simulink model "SimulationEchantillinnesClampingMCC_Simplified"  (R2018b)
settings: Solver=VariableStepAuto  StartTime=0.0  StopTime=2  MaxStep=Ts_elec  RelTol=1e-3
values from neighbouring files (symbols this model uses):
  Imax = Inom    (= 4.4)    [DataMCCEchant.m]
  Kelec = -place(Ae,Be,Pole_elec_desiree)    [DataMCCEchant.m]
  Kmeca = place(Am,Bm,Pole_meca_desiree)    [DataMCCEchant.m]
  Vmax = Vdc    (= 24)    [DataMCCEchant.m]
undefined symbols (not defined in the file or in its folder): DiscIntNeverNeededParam
libraries: simulink x3
settings Model: Creator=romaindelpoux  LastModifiedBy=rdelpoux
settings SolverCC: ZeroCrossControl=DisableAll  AlgebraicLoopSolver=LineSearch
settings SFSimCC: SimUseLocalCustomCode=off
settings RTWCC: RTWUseLocalCustomCode=off

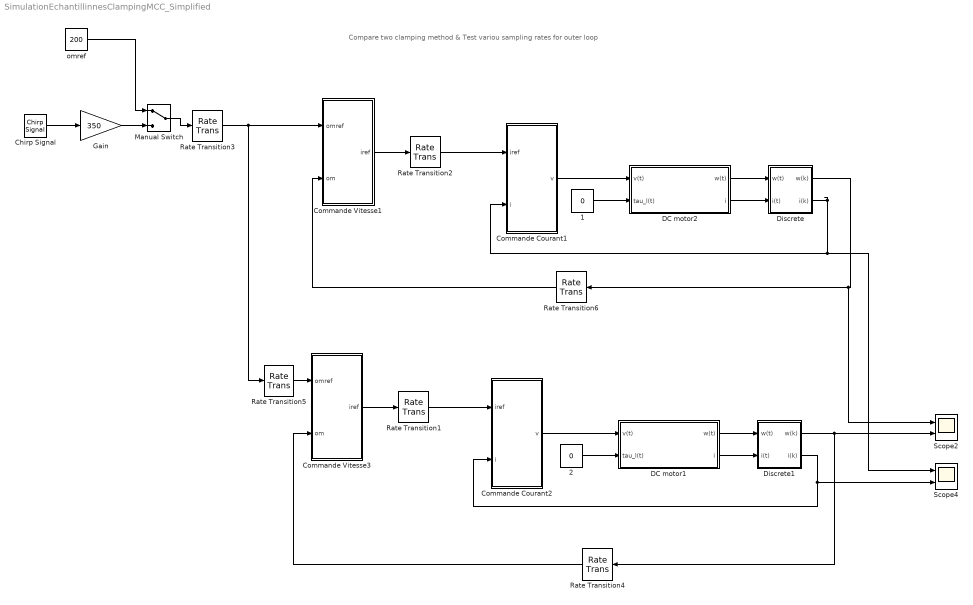
== system SimulationEchantillinnesClampingMCC_Simplified ==
  note: Compare two clamping method
      | & Test variou sampling rates for outer loop
  " 2" : Constant  Value=0
  1 : Constant  Value=0
  Chirp Signal : simulink/Sources/Chirp Signal  f1=0.1  T=20  f2=5
  Commande Courant1 : Subsystem
  Commande Courant2 : Subsystem
  Commande Vitesse1 : Subsystem
  Commande Vitesse3 : Subsystem
  DC motor1 : Subsystem  mask{R=1.22, L=0.0027, Kphi=0.061, J=0.22e-3, F=.0001, C0=0}
      mask prompts: R "Resistance (R) in Ohms"; L "Inductance (L) in H"; Kphi "Back EMF (Kphi) in V/rad/s"; J "J in kgm²"; F "F in N/rad/s"
      mask DialogControl Container3 Prompt: Electrical Parameters
      mask DialogControl Container3_copy Prompt: Mechanical Parameters
  DC motor2 : Subsystem  mask{R=1.22, L=0.0027, Kphi=0.061, J=0.22e-3, F=.0001, C0=0}
      mask prompts: R "Resistance (R) in Ohms"; L "Inductance (L) in H"; Kphi "Back EMF (Kphi) in V/rad/s"; J "J in kgm²"; F "F in N/rad/s"
      mask DialogControl Container3 Prompt: Electrical Parameters
      mask DialogControl Container3_copy Prompt: Mechanical Parameters
  Discrete : Subsystem
  Discrete1 : Subsystem
  Gain : Gain  Gain=350  OutDataTypeStr=Inherit: Inherit via back propagation
  Manual Switch : ManualSwitch
  Rate Transition1 : RateTransition  Deterministic=off  OutPortSampleTime=50e-6
  Rate Transition2 : RateTransition  Deterministic=off  OutPortSampleTime=50e-6
  Rate Transition3 : RateTransition  Deterministic=off  OutPortSampleTime=.002
  Rate Transition4 : RateTransition  Deterministic=off  OutPortSampleTime=0.002
  Rate Transition5 : RateTransition  Deterministic=off
  Rate Transition6 : RateTransition  Deterministic=off  OutPortSampleTime=0.002
  Scope2 : Scope  NumInputPorts=2
  Scope4 : Scope  NumInputPorts=2
  omref : Constant  Value=200  OutDataTypeStr=Inherit: Inherit via back propagation
  wires:
  Chirp Signal/1 -> Gain/1
  Rate Transition2/1 -> Commande Courant1/1(iref)
  DC motor2/1(w(t)) -> Discrete/1(w(t))
  DC motor2/2(i) -> Discrete/2(i(t))
  Discrete/1(w(k)) -> Scope2/1, Rate Transition6/1
  1/1 -> DC motor2/2(tau_l(t))
  Commande Vitesse1/1(iref) -> Rate Transition2/1
  Commande Courant1/1(v) -> DC motor2/1(v(t))
  Gain/1 -> Manual Switch/2
  Manual Switch/1 -> Rate Transition3/1
  omref/1 -> Manual Switch/1
  Rate Transition3/1 -> Rate Transition5/1, Commande Vitesse1/1(omref)
  Commande Courant2/1(v) -> DC motor1/1(v(t))
  Commande Vitesse3/1(iref) -> Rate Transition1/1
  " 2"/1 -> DC motor1/2(tau_l(t))
  Discrete1/1(w(k)) -> Scope2/2, Rate Transition4/1
  DC motor1/1(w(t)) -> Discrete1/1(w(t))
  DC motor1/2(i) -> Discrete1/2(i(t))
  Rate Transition1/1 -> Commande Courant2/1(iref)
  Discrete1/2(i(k)) -> Scope4/2, Commande Courant2/2(i)
  Rate Transition5/1 -> Commande Vitesse3/1(omref)
  Rate Transition4/1 -> Commande Vitesse3/2(om)
  Discrete/2(i(k)) -> Scope4/1, Commande Courant1/2(i)
  Rate Transition6/1 -> Commande Vitesse1/2(om)

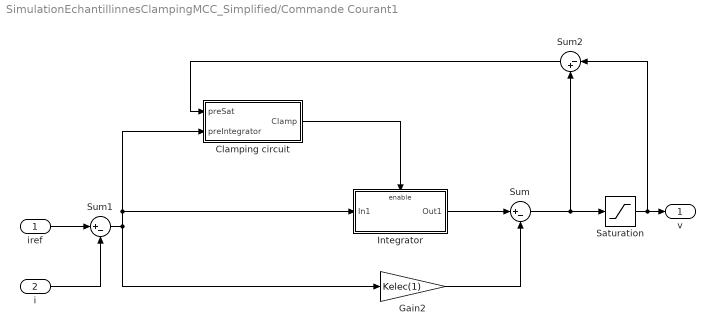
== system SimulationEchantillinnesClampingMCC_Simplified/Commande Courant1 ==
  iref : Inport
  i : Inport  Port=2
  Clamping circuit : Subsystem
  Gain2 : Gain  Gain=Kelec(1)
  Integrator : Subsystem
  Saturation : Saturate  UpperLimit=Vmax  LowerLimit=-Vmax
  Sum : Sum  Inputs=|+-
  Sum1 : Sum  Inputs=|+-
  Sum2 : Sum  Inputs=|-+  OutDataTypeStr=Inherit: Same as accumulator
  v : Outport
  wires:
  Gain2/1 -> Sum/2
  i/1 -> Sum1/2
  iref/1 -> Sum1/1
  Sum1/1 -> Clamping circuit/2(preIntegrator), Integrator/1(In1), Gain2/1
  Clamping circuit/1(Clamp) -> Integrator/Enable
  Sum/1 -> Sum2/2, Saturation/1
  Sum2/1 -> Clamping circuit/1(preSat)
  Saturation/1 -> Sum2/1, v/1
  Integrator/1(Out1) -> Sum/1

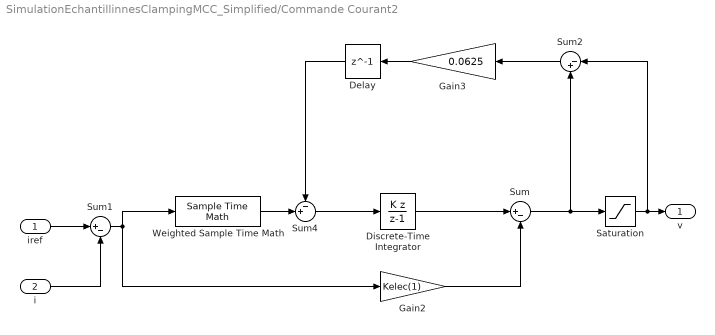
== system SimulationEchantillinnesClampingMCC_Simplified/Commande Courant2 ==
  iref : Inport
  i : Inport  Port=2
  Delay : Delay  DelayLength=1  InitialCondition=0
  Discrete-Time Integrator : DiscreteIntegrator  IntegratorMethod=Accumulation: Backward Euler  SampleTime=-1  ICPrevOutput=DiscIntNeverNeededParam  ICPrevScaledInput=DiscIntNeverNeededParam
  Gain2 : Gain  Gain=Kelec(1)
  Gain3 : Gain  Gain=0.0625
  Saturation : Saturate  UpperLimit=Vmax  LowerLimit=-Vmax
  Sum : Sum  Inputs=|+-
  Sum1 : Sum  Inputs=|+-
  Sum2 : Sum  Inputs=|-+  OutDataTypeStr=Inherit: Same as accumulator
  Sum4 : Sum  Inputs=-+|
  Weighted Sample Time Math : SampleTimeMath  TsampMathOp=*  weightValue=Kelec(2)  TsampMathImp=Offline Scaling Adjustment
  v : Outport
  wires:
  Saturation/1 -> v/1, Sum2/1
  Sum/1 -> Saturation/1, Sum2/2
  iref/1 -> Sum1/1
  i/1 -> Sum1/2
  Gain2/1 -> Sum/2
  Sum1/1 -> Gain2/1, Weighted Sample Time Math/1
  Sum4/1 -> Discrete-Time Integrator/1
  Gain3/1 -> Delay/1
  Delay/1 -> Sum4/1
  Discrete-Time Integrator/1 -> Sum/1
  Sum2/1 -> Gain3/1
  Weighted Sample Time Math/1 -> Sum4/2

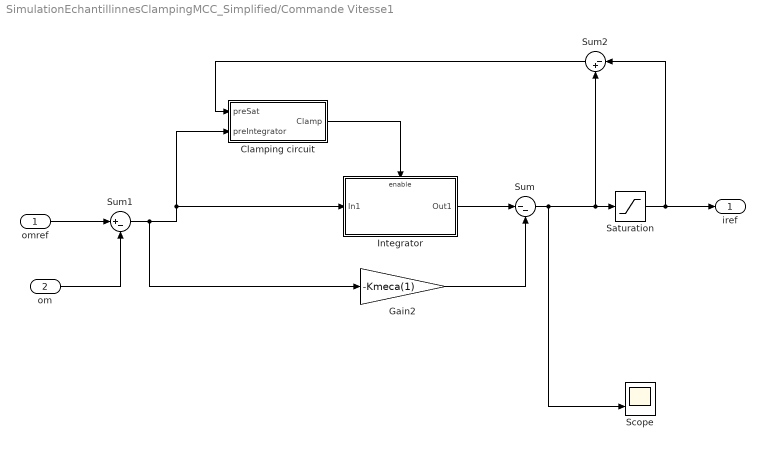
== system SimulationEchantillinnesClampingMCC_Simplified/Commande Vitesse1 ==
  omref : Inport
  om : Inport  Port=2
  Clamping circuit : Subsystem
  Gain2 : Gain  Gain=-Kmeca(1)
  Integrator : Subsystem
  Saturation : Saturate  UpperLimit=Imax  LowerLimit=-Imax
  Scope : Scope  NumInputPorts=2
  Sum : Sum  Inputs=|--
  Sum1 : Sum  Inputs=|+-
  Sum2 : Sum  Inputs=|-+  OutDataTypeStr=Inherit: Same as accumulator
  iref : Outport
  wires:
  Saturation/1 -> Sum2/1, iref/1
  Sum/1 -> Sum2/2, Saturation/1, Scope/2
  om/1 -> Sum1/2
  Gain2/1 -> Sum/2
  omref/1 -> Sum1/1
  Sum2/1 -> Clamping circuit/1(preSat)
  Sum1/1 -> Clamping circuit/2(preIntegrator), Integrator/1(In1), Gain2/1
  Integrator/1(Out1) -> Sum/1
  Clamping circuit/1(Clamp) -> Integrator/Enable

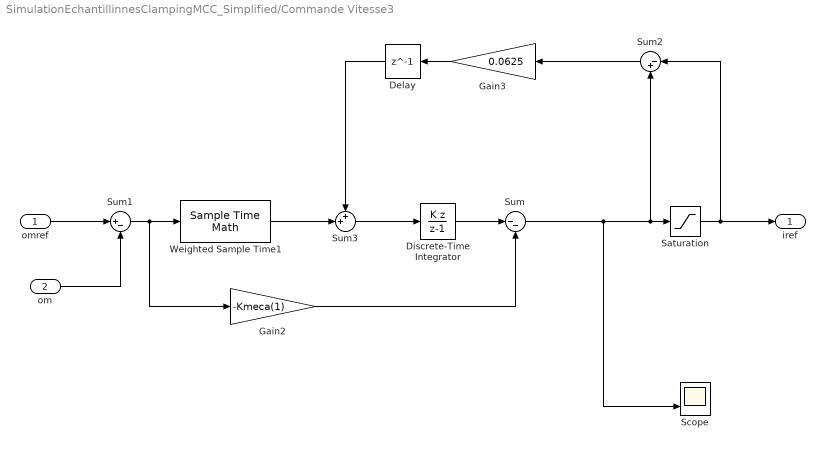
== system SimulationEchantillinnesClampingMCC_Simplified/Commande Vitesse3 ==
  omref : Inport
  om : Inport  Port=2
  Delay : Delay  DelayLength=1  InitialCondition=0
  Discrete-Time Integrator : DiscreteIntegrator  IntegratorMethod=Accumulation: Backward Euler  SampleTime=-1  ICPrevOutput=DiscIntNeverNeededParam  ICPrevScaledInput=DiscIntNeverNeededParam
  Gain2 : Gain  Gain=-Kmeca(1)
  Gain3 : Gain  Gain=0.0625
  Saturation : Saturate  UpperLimit=Imax  LowerLimit=-Imax
  Scope : Scope  NumInputPorts=2
  Sum : Sum  Inputs=|--
  Sum1 : Sum  Inputs=|+-
  Sum2 : Sum  Inputs=|-+  OutDataTypeStr=Inherit: Same as accumulator
  Sum3 : Sum  Inputs=++|
  Weighted Sample Time1 : SampleTimeMath  TsampMathOp=*  weightValue=Kmeca(2)
  iref : Outport
  wires:
  Delay/1 -> Sum3/1
  Gain3/1 -> Delay/1
  Sum3/1 -> Discrete-Time Integrator/1
  Discrete-Time Integrator/1 -> Sum/1
  Saturation/1 -> iref/1, Sum2/1
  Sum/1 -> Scope/2, Sum2/2, Saturation/1
  om/1 -> Sum1/2
  omref/1 -> Sum1/1
  Sum2/1 -> Gain3/1
  Gain2/1 -> Sum/2
  Sum1/1 -> Weighted Sample Time1/1, Gain2/1
  Weighted Sample Time1/1 -> Sum3/2

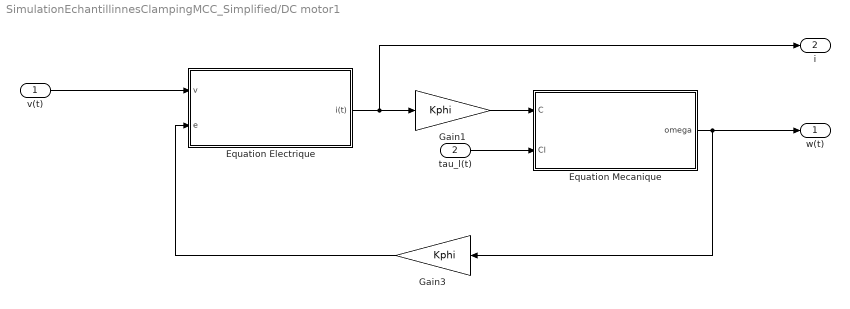
== system SimulationEchantillinnesClampingMCC_Simplified/DC motor1 ==
  v(t) : Inport
  tau_l(t) : Inport  Port=2
  Equation Electrique : Subsystem
  Equation Mecanique : Subsystem
  Gain1 : Gain  Gain=Kphi
  "Gain3  " : Gain  Gain=Kphi
  w(t) : Outport
  i : Outport  Port=2
  wires:
  "Gain3  "/1 -> Equation Electrique/2(e)
  Gain1/1 -> Equation Mecanique/1(C)
  tau_l(t)/1 -> Equation Mecanique/2(Cl)
  Equation Electrique/1(i(t)) -> i/1, Gain1/1
  Equation Mecanique/1(omega) -> w(t)/1, "Gain3  "/1
  v(t)/1 -> Equation Electrique/1(v)

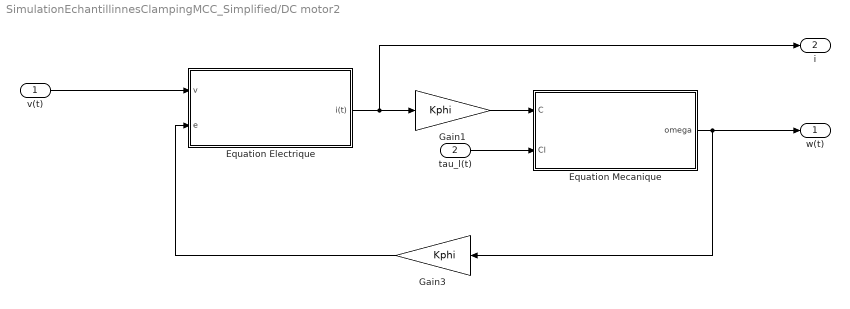
== system SimulationEchantillinnesClampingMCC_Simplified/DC motor2 ==
  v(t) : Inport
  tau_l(t) : Inport  Port=2
  Equation Electrique : Subsystem
  Equation Mecanique : Subsystem
  Gain1 : Gain  Gain=Kphi
  "Gain3  " : Gain  Gain=Kphi
  w(t) : Outport
  i : Outport  Port=2
  wires:
  v(t)/1 -> Equation Electrique/1(v)
  Equation Mecanique/1(omega) -> "Gain3  "/1, w(t)/1
  Equation Electrique/1(i(t)) -> Gain1/1, i/1
  tau_l(t)/1 -> Equation Mecanique/2(Cl)
  Gain1/1 -> Equation Mecanique/1(C)
  "Gain3  "/1 -> Equation Electrique/2(e)

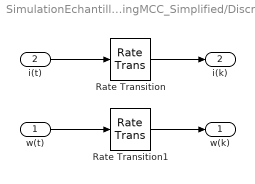
== system SimulationEchantillinnesClampingMCC_Simplified/Discrete ==
  w(t) : Inport
  i(t) : Inport  Port=2
  Rate Transition : RateTransition  Deterministic=off  OutPortSampleTime=50e-6
  Rate Transition1 : RateTransition  Deterministic=off  OutPortSampleTime=.002
  w(k) : Outport
  i(k) : Outport  Port=2
  wires:
  w(t)/1 -> Rate Transition1/1
  i(t)/1 -> Rate Transition/1
  Rate Transition1/1 -> w(k)/1
  Rate Transition/1 -> i(k)/1

== system SimulationEchantillinnesClampingMCC_Simplified/Discrete1 ==
  w(t) : Inport
  i(t) : Inport  Port=2
  Rate Transition : RateTransition  Deterministic=off  OutPortSampleTime=50e-6
  Rate Transition1 : RateTransition  Deterministic=off  OutPortSampleTime=.002
  w(k) : Outport
  i(k) : Outport  Port=2
  wires:
  Rate Transition/1 -> i(k)/1
  Rate Transition1/1 -> w(k)/1
  i(t)/1 -> Rate Transition/1
  w(t)/1 -> Rate Transition1/1

== system SimulationEchantillinnesClampingMCC_Simplified/Commande Courant1/Clamping circuit ==
  note: La logique de clamping permet de bloquer l'entée de l'action intégrale.
      | Ainsi, si la sortie du controlleur est en dehors des limites imposés (saturée), alors l'action intégrale du correcteur est verrouyé (clamping).
      | L'action intégrale est verroullé si la sortie du correcteur (commande) est en dehors des saturations et que le signe de cette sortie est égale
      | à l'entrée du signal à intégrer.
  preSat : Inport  DisableCoverage=on
  preIntegrator : Inport  DisableCoverage=on  Port=2
  Compare To Zero1 : simulink/Logic and Bit Operations/Compare To Zero  relop=<=  OutDataTypeStr=boolean
  Delay : Delay  DelayLength=1  InitialCondition=0
  Multiply : Product
  Clamp : Outport  DisableCoverage=on
  wires:
  Compare To Zero1/1 -> Clamp/1
  preIntegrator/1 -> Multiply/2
  Multiply/1 -> Compare To Zero1/1
  preSat/1 -> Delay/1
  Delay/1 -> Multiply/1

== system SimulationEchantillinnesClampingMCC_Simplified/Commande Courant1/Integrator ==
  In1 : Inport
  Enable : EnablePort
  Discrete-Time Integrator : DiscreteIntegrator  SampleTime=50e-6  ICPrevOutput=DiscIntNeverNeededParam  ICPrevScaledInput=DiscIntNeverNeededParam
  Gain1 : Gain  Gain=Kelec(2)
  Out1 : Outport
  wires:
  Discrete-Time Integrator/1 -> Gain1/1
  In1/1 -> Discrete-Time Integrator/1
  Gain1/1 -> Out1/1

== system SimulationEchantillinnesClampingMCC_Simplified/Commande Vitesse1/Clamping circuit ==
  note: La logique de clamping permet de bloquer l'entée de l'action intégrale.
      | Ainsi, si la sortie du controlleur est en dehors des limites imposés (saturée), alors l'action intégrale du correcteur est verrouyé (clamping).
      | L'action intégrale est verroullé si la sortie du correcteur (commande) est en dehors des saturations et que le signe de cette sortie est égale
      | à l'entrée du signal à intégrer.
  preSat : Inport  DisableCoverage=on
  preIntegrator : Inport  DisableCoverage=on  Port=2
  Compare To Zero1 : simulink/Logic and Bit Operations/Compare To Zero  relop=<=  OutDataTypeStr=boolean
  Delay : Delay  DelayLength=1  InitialCondition=0
  Multiply : Product
  Clamp : Outport  DisableCoverage=on
  wires:
  Compare To Zero1/1 -> Clamp/1
  preIntegrator/1 -> Multiply/2
  Multiply/1 -> Compare To Zero1/1
  preSat/1 -> Delay/1
  Delay/1 -> Multiply/1

== system SimulationEchantillinnesClampingMCC_Simplified/Commande Vitesse1/Integrator ==
  In1 : Inport
  Enable : EnablePort
  Discrete-Time Integrator : DiscreteIntegrator  SampleTime=-1  ICPrevOutput=DiscIntNeverNeededParam  ICPrevScaledInput=DiscIntNeverNeededParam
  Gain1 : Gain  Gain=Kmeca(2)
  Out1 : Outport
  wires:
  Discrete-Time Integrator/1 -> Gain1/1
  Gain1/1 -> Out1/1
  In1/1 -> Discrete-Time Integrator/1

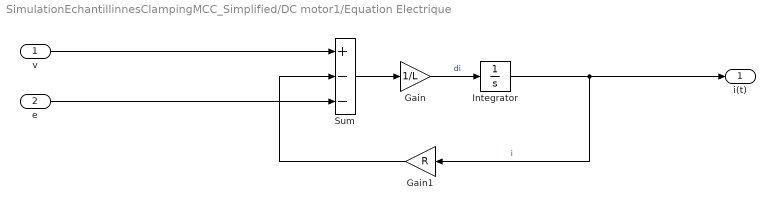
== system SimulationEchantillinnesClampingMCC_Simplified/DC motor1/Equation Electrique ==
  v : Inport
  e : Inport  Port=2
  Gain : Gain  Gain=1/L
  Gain1 : Gain  Gain=R
  Integrator : Integrator
  Sum : Sum  Inputs=+--
  i(t) : Outport
  wires:
  Gain1/1 -> Sum/2
  Sum/1 -> Gain/1
  Integrator/1 -> i(t)/1, Gain1/1  "i"
  Gain/1 -> Integrator/1  "di"
  v/1 -> Sum/1
  e/1 -> Sum/3

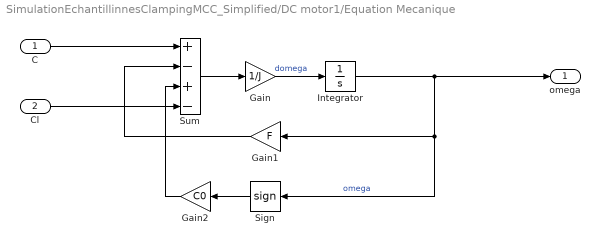
== system SimulationEchantillinnesClampingMCC_Simplified/DC motor1/Equation Mecanique ==
  C : Inport
  Cl : Inport  Port=2
  Gain : Gain  Gain=1/J
  Gain1 : Gain  Gain=F
  Gain2 : Gain  Gain=C0
  Integrator : Integrator
  Sign : Signum
  Sum : Sum  Inputs=+-+-
  omega : Outport
  wires:
  Gain/1 -> Integrator/1  "domega"
  Integrator/1 -> Sign/1, Gain1/1, omega/1  "omega"
  Sum/1 -> Gain/1
  Gain1/1 -> Sum/2
  Sign/1 -> Gain2/1
  Gain2/1 -> Sum/3
  C/1 -> Sum/1
  Cl/1 -> Sum/4

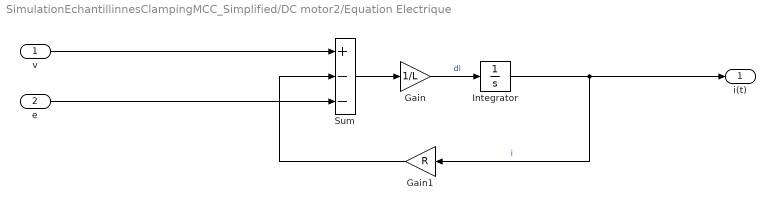
== system SimulationEchantillinnesClampingMCC_Simplified/DC motor2/Equation Electrique ==
  v : Inport
  e : Inport  Port=2
  Gain : Gain  Gain=1/L
  Gain1 : Gain  Gain=R
  Integrator : Integrator
  Sum : Sum  Inputs=+--
  i(t) : Outport
  wires:
  e/1 -> Sum/3
  v/1 -> Sum/1
  Gain/1 -> Integrator/1  "di"
  Integrator/1 -> Gain1/1, i(t)/1  "i"
  Sum/1 -> Gain/1
  Gain1/1 -> Sum/2

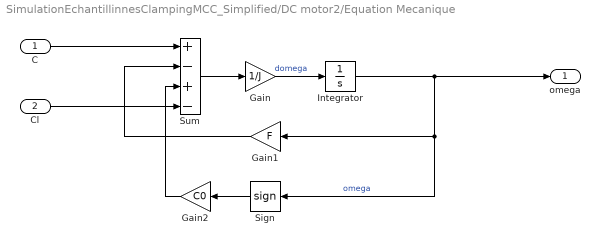
== system SimulationEchantillinnesClampingMCC_Simplified/DC motor2/Equation Mecanique ==
  C : Inport
  Cl : Inport  Port=2
  Gain : Gain  Gain=1/J
  Gain1 : Gain  Gain=F
  Gain2 : Gain  Gain=C0
  Integrator : Integrator
  Sign : Signum
  Sum : Sum  Inputs=+-+-
  omega : Outport
  wires:
  Cl/1 -> Sum/4
  C/1 -> Sum/1
  Gain2/1 -> Sum/3
  Sign/1 -> Gain2/1
  Gain1/1 -> Sum/2
  Sum/1 -> Gain/1
  Integrator/1 -> omega/1, Gain1/1, Sign/1  "omega"
  Gain/1 -> Integrator/1  "domega"
